simulink model "sFlow_Raul"  (R2017a)
settings: Solver=VariableStepAuto  StartTime=0.0  StopTime=0.2  MaxStep=1e-6  RelTol=1e-3
values from neighbouring files (symbols this model uses):
  H1 = tf(n11,d11)    [funcionestransf.m]
  H2 = tf(n12,d12)    [funcionestransf.m]
libraries: simulink_extras x2, powerlib_meascontrol x1
settings Model: Creator=erich  LastModifiedBy=erich

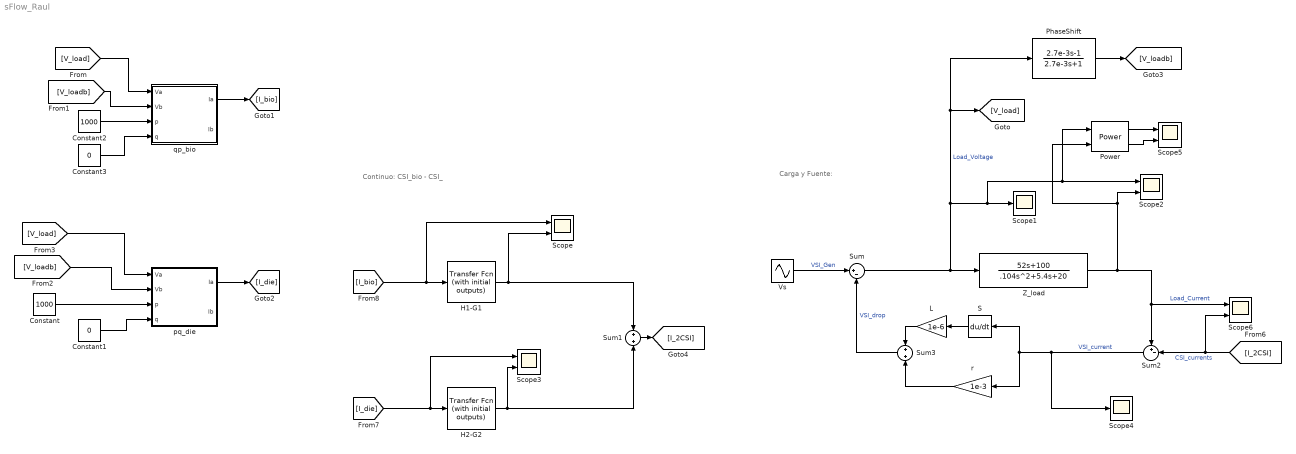
== system sFlow_Raul ==
  note: Continuo: CSI_bio - CSI_
  note: Carga y Fuente:
  Constant : Constant  Value=1000
  Constant1 : Constant  Value=0
  Constant2 : Constant  Value=1000
  Constant3 : Constant  Value=0
  H1-G1 : simulink_extras/Additional Linear/Transfer Fcn (with initial outputs)  N=H1.Numerator{1}  D=H1.Denominator{1}  Y0=0  U0=0
  H2-G2 : simulink_extras/Additional Linear/Transfer Fcn (with initial outputs)  N=H2.Numerator{1}  D=H2.Denominator{1}  Y0=0  U0=0
  L : Gain  Gain=1e-6
  PhaseShift : TransferFcn  Numerator=[2.7e-3 -1]  Denominator=[2.7e-3 1]
  Power : powerlib_meascontrol/Measurements/Power  Freq=60  Vinit=[1, 0]  Iinit=[1, 0]  Ts=0
      settings: SourceProductName=Simscape Power Systems
  S : Derivative  CoefficientInTFapproximation=1e-4
  Scope{,2..3,5..6} (5 alike) : Scope  NumInputPorts=2
  Scope1 : Scope
  Scope4 : Scope
  Sum : Sum  Inputs=|+-
  Sum1 : Sum  Inputs=+|+
  Sum2 : Sum  Inputs=+-|
  Sum3 : Sum  Inputs=+|+
  Vs : Sin  Amplitude=170  Frequency=2*pi*60  SampleTime=0
  Z_load : TransferFcn  Numerator=[52 100]  Denominator=[.104 5.4 20]
  pq_die : MATLAB Function  TreatAsAtomicUnit=on
  qp_bio : MATLAB Function  TreatAsAtomicUnit=on
  r : Gain  Gain=1e-3
  wires:
  [I_bio] -> Scope/1, H1-G1/1
  H1-G1/1 -> Sum1/1, Scope/2
  H2-G2/1 -> Scope3/2, Sum1/2
  [I_die] -> Scope3/1, H2-G2/1
  qp_bio/1(Ia) -> [I_bio]
  pq_die/1(Ia) -> [I_die]
  Constant/1 -> pq_die/3(p)
  Constant1/1 -> pq_die/4(q)
  Constant3/1 -> qp_bio/4(q)
  Constant2/1 -> qp_bio/3(p)
  Vs/1 -> Sum/1  "VSI_Gen"
  Sum/1 -> PhaseShift/1, [V_load], Power/1, Scope2/1, Scope1/1, Z_load/1  "Load_Voltage"
  Sum3/1 -> Sum/2  "VSI_drop"
  Z_load/1 -> Power/2, Scope2/2, Scope6/1, Sum2/1  "Load_Current"
  Sum1/1 -> [I_2CSI]
  [I_2CSI] -> Scope6/2, Sum2/2  "CSI_currents"
  Sum2/1 -> Scope4/1, r/1, S/1  "VSI_current"
  S/1 -> L/1
  r/1 -> Sum3/2
  L/1 -> Sum3/1
  PhaseShift/1 -> [V_loadb]
  Power/1 -> Scope5/1
  Power/2 -> Scope5/2
  [V_loadb] -> pq_die/2(Vb)
  [V_load] -> pq_die/1(Va)
  [V_loadb] -> qp_bio/2(Vb)
  [V_load] -> qp_bio/1(Va)

== matlab function sFlow_Raul/pq_die ==
  data: Va input; Ia output; Vb input; p input; q input; Ib output
function [Ia, Ib] = fcn(Va, Vb, p, q)
%#codegen

% divide by zero protection
if(abs((Va^2+Vb^2))<=1000*eps(0))
    det = 1/eps(0);
else
    det = 1/(Va^2+Vb^2); % constante auxiliar
end;
%det = 1/(Va^2+Vb^2);

Mat = det*[Va Vb; Vb -Va];
Iab = Mat*[2*p;2*q];

Iaaux = Iab(1);
Ibaux = Iab(2);

ilim=1e3;

if(Iaaux>ilim)
    Iaaux=ilim;
end;
if(Iaaux<-ilim)
    Iaaux =-ilim;    
end;

if(isnan(Iaaux))
    Iaaux=0;
end;
%-----------------


if(Ibaux>ilim)
    Ibaux=ilim;
end;
if(Ibaux<-ilim)
    Ibaux =-ilim;    
end;

if(isnan(Ibaux))
    Ibaux=0;
end;
%-----------------


Ia = Iaaux;
Ib = Ibaux;

== matlab function sFlow_Raul/qp_bio ==
  data: Va input; Ia output; Vb input; p input; q input; Ib output
function [Ia, Ib] = fcn(Va, Vb, p, q)
%#codegen

% divide by zero protection
if(abs((Va^2+Vb^2))<=1000*eps(0))
    det = 1/eps(0);
else
    det = 1/(Va^2+Vb^2); % constante auxiliar
end;
%det = 1/(Va^2+Vb^2);

Mat = det*[Va Vb; Vb -Va];
Iab = Mat*[2*p;2*q];

Iaaux = Iab(1);
Ibaux = Iab(2);

ilim=1e3;

if(Iaaux>ilim)
    Iaaux=ilim;
end;
if(Iaaux<-ilim)
    Iaaux =-ilim;    
end;

if(isnan(Iaaux))
    Iaaux=0;
end;
%-----------------


if(Ibaux>ilim)
    Ibaux=ilim;
end;
if(Ibaux<-ilim)
    Ibaux =-ilim;    
end;

if(isnan(Ibaux))
    Ibaux=0;
end;
%-----------------


Ia = Iaaux;
Ib = Ibaux;
